simulink model "gm_uz_axi_testIP"  (R2020b)
settings: Solver=FixedStepDiscrete  StartTime=0.0  StopTime=10.0  RelTol=1e-3
settings Model: Creator=ts  LastModifiedBy=ts
settings DataIOCC: LimitDataPoints=on  SaveOutput=off  SaveTime=off
settings OptimizationCC: BlockReduction=off  ConditionallyExecuteInputs=off  DefaultParameterBehavior=Inlined  LifeSpan=inf
settings DebuggingCC: AlgebraicLoopMsg=error  InheritedTsInSrcMsg=none  SingleTaskRateTransMsg=error  AllowSymbolicDim=off  StrictBusMsg=ErrorOnBusTreatedAsVector  SFUnexpectedBacktrackingDiag=warning  SFNoUnconditionalDefaultTransitionDiag=warning  SFExecutionAtInitializationDiag=none  ArithmeticOperatorsInVariantConditions=warning
settings HardwareCC: ProdBitPerPointer=32  ProdBitPerSizeT=32  ProdBitPerPtrDiffT=32  ProdLargestAtomicFloat=None  ProdIntDivRoundTo=Undefined  ProdEndianess=Unspecified  ProdWordSize=32  ProdHWDeviceType=ASIC/FPGA->ASIC/FPGA  ProdEqTarget=off
settings SFSimCC: SimUseLocalCustomCode=off  CustomCodeUndefinedFunction=UseInterfaceOnly
settings RTWCC: RTWUseLocalCustomCode=off
settings CodeAppCC: StateflowObjectComments=on
settings GRTTargetCC: TargetLangStandard=C89/C90 (ANSI)
settings ConfigComp: CovScope=ReferencedModels  CovMetricSettings=dw  CovSaveCumulativeToWorkspaceVar=on  CovSaveSingleToWorkspaceVar=on  CovExternalEMLEnable=off  CovSFcnEnable=off

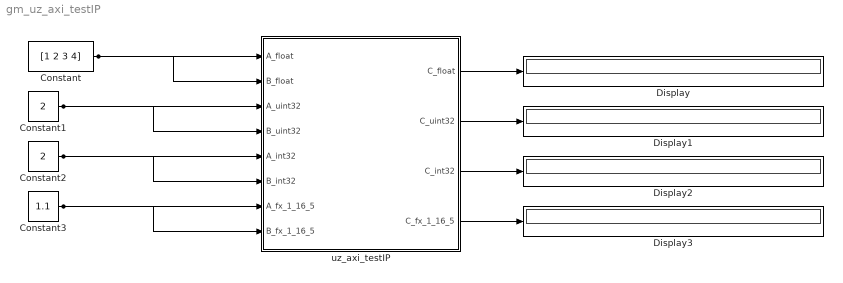
== system gm_uz_axi_testIP ==
  Constant : Constant  Value=[1 2 3 4]  OutDataTypeStr=single  SampleTime=-1
  Constant1 : Constant  Value=2  OutDataTypeStr=uint32  SampleTime=-1
  Constant2 : Constant  Value=2  OutDataTypeStr=int32  SampleTime=-1
  Constant3 : Constant  Value=1.1  OutDataTypeStr=fixdt(1,16,5)  SampleTime=-1
  Display{,1..3} (4 alike) : Display
  uz_axi_testIP : Subsystem  TreatAsAtomicUnit=on
  wires:
  Constant3/1 -> uz_axi_testIP/7(A_fx_1_16_5), uz_axi_testIP/8(B_fx_1_16_5)
  Constant2/1 -> uz_axi_testIP/5(A_int32), uz_axi_testIP/6(B_int32)
  uz_axi_testIP/4(C_fx_1_16_5) -> Display3/1
  uz_axi_testIP/3(C_int32) -> Display2/1
  uz_axi_testIP/2(C_uint32) -> Display1/1
  Constant1/1 -> uz_axi_testIP/3(A_uint32), uz_axi_testIP/4(B_uint32)
  uz_axi_testIP/1(C_float) -> Display/1
  Constant/1 -> uz_axi_testIP/1(A_float), uz_axi_testIP/2(B_float)

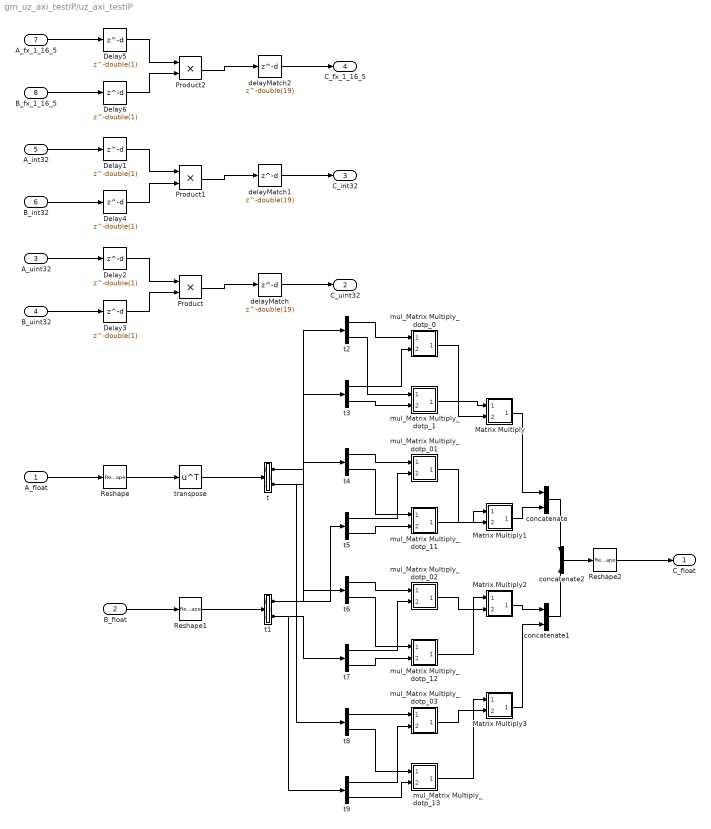
== system gm_uz_axi_testIP/uz_axi_testIP ==
  A_float : Inport  OutDataTypeStr=single  PortDimensions=[4]  SampleTime=0.2
  B_float : Inport  Port=2  OutDataTypeStr=single  PortDimensions=[4]  SampleTime=0.2
  A_uint32 : Inport  Port=3  OutDataTypeStr=uint32  PortDimensions=1  SampleTime=0.2
  B_uint32 : Inport  Port=4  OutDataTypeStr=uint32  PortDimensions=1  SampleTime=0.2
  A_int32 : Inport  Port=5  OutDataTypeStr=int32  PortDimensions=1  SampleTime=0.2
  B_int32 : Inport  Port=6  OutDataTypeStr=int32  PortDimensions=1  SampleTime=0.2
  A_fx_1_16_5 : Inport  Port=7  OutDataTypeStr=fixdt(1, 16, 5)  PortDimensions=1  SampleTime=0.2
  B_fx_1_16_5 : Inport  Port=8  OutDataTypeStr=fixdt(1, 16, 5)  PortDimensions=1  SampleTime=0.2
  Delay{1..6} (6 alike) : Delay  DelayLength=double(1)  InitialCondition=0  SampleTime=0.2
  Matrix Multiply : Subsystem
      mask Display: disp('NFP\nadd');
  Matrix Multiply1 : Subsystem
      mask Display: disp('NFP\nadd');
  Matrix Multiply2 : Subsystem
      mask Display: disp('NFP\nadd');
  Matrix Multiply3 : Subsystem
      mask Display: disp('NFP\nadd');
  Product : Product  Inputs=**  OutDataTypeStr=uint32  SampleTime=0.2
  Product1 : Product  Inputs=**  OutDataTypeStr=int32  SampleTime=0.2
  Product2 : Product  Inputs=**  OutDataTypeStr=fixdt(1, 16, 5)  SampleTime=0.2
  Reshape : Reshape  OutputDimensionality=Customize  OutputDimensions=[2,2]
  Reshape1 : Reshape  OutputDimensionality=Customize  OutputDimensions=[2,2]
  Reshape2 : Reshape  OutputDimensions=[4]
  concatenate : Concatenate
  concatenate1 : Concatenate
  concatenate2 : Concatenate  Mode=Multidimensional array  ConcatenateDimension=2
  delayMatch : Delay  DelayLength=double(19)  InitialCondition=0  SampleTime=0.2
  delayMatch1 : Delay  DelayLength=double(19)  InitialCondition=0  SampleTime=0.2
  delayMatch2 : Delay  DelayLength=double(19)  InitialCondition=0  SampleTime=0.2
  mul_Matrix Multiply_dotp_0 : Subsystem
      mask Display: disp('NFP\nmul');
  mul_Matrix Multiply_dotp_01 : Subsystem
      mask Display: disp('NFP\nmul');
  mul_Matrix Multiply_dotp_02 : Subsystem
      mask Display: disp('NFP\nmul');
  mul_Matrix Multiply_dotp_03 : Subsystem
      mask Display: disp('NFP\nmul');
  mul_Matrix Multiply_dotp_1 : Subsystem
      mask Display: disp('NFP\nmul');
  mul_Matrix Multiply_dotp_11 : Subsystem
      mask Display: disp('NFP\nmul');
  mul_Matrix Multiply_dotp_12 : Subsystem
      mask Display: disp('NFP\nmul');
  mul_Matrix Multiply_dotp_13 : Subsystem
      mask Display: disp('NFP\nmul');
  t : Subsystem
  t1 : Subsystem
  t{2..9} (8 alike) : Demux  Outputs=2
  transpose : Math  Operator=transpose  SaturateOnIntegerOverflow=on
  C_float : Outport  VectorParamsAs1DForOutWhenUnconnected=off
  C_uint32 : Outport  Port=2  VectorParamsAs1DForOutWhenUnconnected=off
  C_int32 : Outport  Port=3  VectorParamsAs1DForOutWhenUnconnected=off
  C_fx_1_16_5 : Outport  Port=4  VectorParamsAs1DForOutWhenUnconnected=off
  wires:
  A_float/1 -> Reshape/1
  B_float/1 -> Reshape1/1
  A_uint32/1 -> Delay2/1
  B_uint32/1 -> Delay3/1
  A_int32/1 -> Delay1/1
  B_int32/1 -> Delay4/1
  A_fx_1_16_5/1 -> Delay5/1
  B_fx_1_16_5/1 -> Delay6/1
  Delay1/1 -> Product1/1
  Delay2/1 -> Product/1
  Delay3/1 -> Product/2
  Delay4/1 -> Product1/2
  Delay5/1 -> Product2/1
  Delay6/1 -> Product2/2
  concatenate2/1 -> Reshape2/1
  delayMatch/1 -> C_uint32/1
  delayMatch1/1 -> C_int32/1
  delayMatch2/1 -> C_fx_1_16_5/1
  Reshape/1 -> transpose/1
  Reshape1/1 -> t1/1(in0)
  Reshape2/1 -> C_float/1
  transpose/1 -> t/1(in0)
  t/1(out0) -> t6/1, t2/1
  t/2(out1) -> t8/1, t4/1
  t1/1(out0) -> t5/1, t3/1
  t1/2(out1) -> t9/1, t7/1
  t2/1 -> mul_Matrix Multiply_dotp_0/1(In1)
  t2/2 -> mul_Matrix Multiply_dotp_1/1(In1)
  t3/1 -> mul_Matrix Multiply_dotp_0/2(In2)
  t3/2 -> mul_Matrix Multiply_dotp_1/2(In2)
  t4/1 -> mul_Matrix Multiply_dotp_01/1(In1)
  t4/2 -> mul_Matrix Multiply_dotp_11/1(In1)
  t5/1 -> mul_Matrix Multiply_dotp_01/2(In2)
  t5/2 -> mul_Matrix Multiply_dotp_11/2(In2)
  concatenate/1 -> concatenate2/1
  t6/1 -> mul_Matrix Multiply_dotp_02/1(In1)
  t6/2 -> mul_Matrix Multiply_dotp_12/1(In1)
  t7/1 -> mul_Matrix Multiply_dotp_02/2(In2)
  t7/2 -> mul_Matrix Multiply_dotp_12/2(In2)
  t8/1 -> mul_Matrix Multiply_dotp_03/1(In1)
  t8/2 -> mul_Matrix Multiply_dotp_13/1(In1)
  t9/1 -> mul_Matrix Multiply_dotp_03/2(In2)
  t9/2 -> mul_Matrix Multiply_dotp_13/2(In2)
  concatenate1/1 -> concatenate2/2
  mul_Matrix Multiply_dotp_0/1(Out1) -> Matrix Multiply/2(In2)
  mul_Matrix Multiply_dotp_1/1(Out1) -> Matrix Multiply/1(In1)
  Matrix Multiply/1(Out1) -> concatenate/1
  mul_Matrix Multiply_dotp_01/1(Out1) -> Matrix Multiply1/2(In2)
  mul_Matrix Multiply_dotp_11/1(Out1) -> Matrix Multiply1/1(In1)
  Matrix Multiply1/1(Out1) -> concatenate/2
  mul_Matrix Multiply_dotp_02/1(Out1) -> Matrix Multiply2/2(In2)
  mul_Matrix Multiply_dotp_12/1(Out1) -> Matrix Multiply2/1(In1)
  Matrix Multiply2/1(Out1) -> concatenate1/1
  mul_Matrix Multiply_dotp_03/1(Out1) -> Matrix Multiply3/2(In2)
  mul_Matrix Multiply_dotp_13/1(Out1) -> Matrix Multiply3/1(In1)
  Matrix Multiply3/1(Out1) -> concatenate1/2
  Product/1 -> delayMatch/1
  Product1/1 -> delayMatch1/1
  Product2/1 -> delayMatch2/1

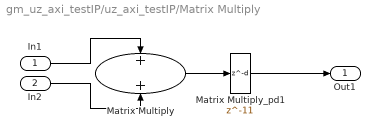
== system gm_uz_axi_testIP/uz_axi_testIP/Matrix Multiply ==
  In1 : Inport
  In2 : Inport  Port=2
  Matrix Multiply : Sum  OutDataTypeStr=single  SampleTime=0.2
  Matrix Multiply_pd1 : Delay  DelayLength=11
  Out1 : Outport
  wires:
  In1/1 -> Matrix Multiply/1
  In2/1 -> Matrix Multiply/2
  Matrix Multiply/1 -> Matrix Multiply_pd1/1
  Matrix Multiply_pd1/1 -> Out1/1

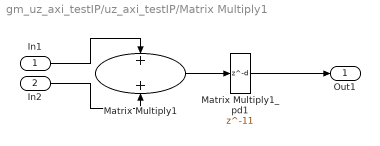
== system gm_uz_axi_testIP/uz_axi_testIP/Matrix Multiply1 ==
  In1 : Inport
  In2 : Inport  Port=2
  Matrix Multiply1 : Sum  OutDataTypeStr=single  SampleTime=0.2
  Matrix Multiply1_pd1 : Delay  DelayLength=11
  Out1 : Outport
  wires:
  In1/1 -> Matrix Multiply1/1
  In2/1 -> Matrix Multiply1/2
  Matrix Multiply1/1 -> Matrix Multiply1_pd1/1
  Matrix Multiply1_pd1/1 -> Out1/1

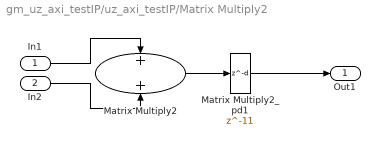
== system gm_uz_axi_testIP/uz_axi_testIP/Matrix Multiply2 ==
  In1 : Inport
  In2 : Inport  Port=2
  Matrix Multiply2 : Sum  OutDataTypeStr=single  SampleTime=0.2
  Matrix Multiply2_pd1 : Delay  DelayLength=11
  Out1 : Outport
  wires:
  In1/1 -> Matrix Multiply2/1
  In2/1 -> Matrix Multiply2/2
  Matrix Multiply2/1 -> Matrix Multiply2_pd1/1
  Matrix Multiply2_pd1/1 -> Out1/1

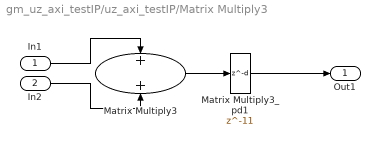
== system gm_uz_axi_testIP/uz_axi_testIP/Matrix Multiply3 ==
  In1 : Inport
  In2 : Inport  Port=2
  Matrix Multiply3 : Sum  OutDataTypeStr=single  SampleTime=0.2
  Matrix Multiply3_pd1 : Delay  DelayLength=11
  Out1 : Outport
  wires:
  In1/1 -> Matrix Multiply3/1
  In2/1 -> Matrix Multiply3/2
  Matrix Multiply3/1 -> Matrix Multiply3_pd1/1
  Matrix Multiply3_pd1/1 -> Out1/1

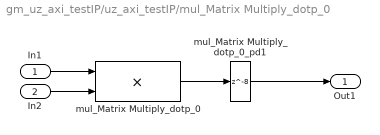
== system gm_uz_axi_testIP/uz_axi_testIP/mul_Matrix Multiply_dotp_0 ==
  In1 : Inport
  In2 : Inport  Port=2
  mul_Matrix Multiply_dotp_0 : Product  Inputs=**  OutDataTypeStr=single  SampleTime=0.2
  mul_Matrix Multiply_dotp_0_pd1 : Delay  DelayLength=8
  Out1 : Outport
  wires:
  In1/1 -> mul_Matrix Multiply_dotp_0/1
  In2/1 -> mul_Matrix Multiply_dotp_0/2
  mul_Matrix Multiply_dotp_0/1 -> mul_Matrix Multiply_dotp_0_pd1/1
  mul_Matrix Multiply_dotp_0_pd1/1 -> Out1/1

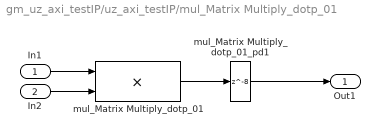
== system gm_uz_axi_testIP/uz_axi_testIP/mul_Matrix Multiply_dotp_01 ==
  In1 : Inport
  In2 : Inport  Port=2
  mul_Matrix Multiply_dotp_01 : Product  Inputs=**  OutDataTypeStr=single  SampleTime=0.2
  mul_Matrix Multiply_dotp_01_pd1 : Delay  DelayLength=8
  Out1 : Outport
  wires:
  In1/1 -> mul_Matrix Multiply_dotp_01/1
  In2/1 -> mul_Matrix Multiply_dotp_01/2
  mul_Matrix Multiply_dotp_01/1 -> mul_Matrix Multiply_dotp_01_pd1/1
  mul_Matrix Multiply_dotp_01_pd1/1 -> Out1/1

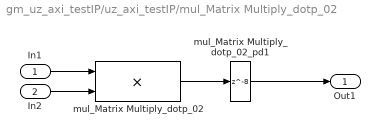
== system gm_uz_axi_testIP/uz_axi_testIP/mul_Matrix Multiply_dotp_02 ==
  In1 : Inport
  In2 : Inport  Port=2
  mul_Matrix Multiply_dotp_02 : Product  Inputs=**  OutDataTypeStr=single  SampleTime=0.2
  mul_Matrix Multiply_dotp_02_pd1 : Delay  DelayLength=8
  Out1 : Outport
  wires:
  In1/1 -> mul_Matrix Multiply_dotp_02/1
  In2/1 -> mul_Matrix Multiply_dotp_02/2
  mul_Matrix Multiply_dotp_02/1 -> mul_Matrix Multiply_dotp_02_pd1/1
  mul_Matrix Multiply_dotp_02_pd1/1 -> Out1/1

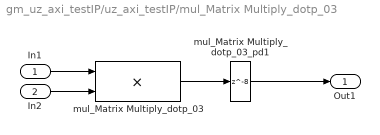
== system gm_uz_axi_testIP/uz_axi_testIP/mul_Matrix Multiply_dotp_03 ==
  In1 : Inport
  In2 : Inport  Port=2
  mul_Matrix Multiply_dotp_03 : Product  Inputs=**  OutDataTypeStr=single  SampleTime=0.2
  mul_Matrix Multiply_dotp_03_pd1 : Delay  DelayLength=8
  Out1 : Outport
  wires:
  In1/1 -> mul_Matrix Multiply_dotp_03/1
  In2/1 -> mul_Matrix Multiply_dotp_03/2
  mul_Matrix Multiply_dotp_03/1 -> mul_Matrix Multiply_dotp_03_pd1/1
  mul_Matrix Multiply_dotp_03_pd1/1 -> Out1/1

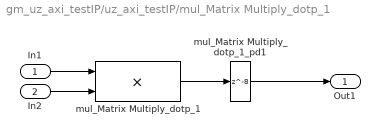
== system gm_uz_axi_testIP/uz_axi_testIP/mul_Matrix Multiply_dotp_1 ==
  In1 : Inport
  In2 : Inport  Port=2
  mul_Matrix Multiply_dotp_1 : Product  Inputs=**  OutDataTypeStr=single  SampleTime=0.2
  mul_Matrix Multiply_dotp_1_pd1 : Delay  DelayLength=8
  Out1 : Outport
  wires:
  In1/1 -> mul_Matrix Multiply_dotp_1/1
  In2/1 -> mul_Matrix Multiply_dotp_1/2
  mul_Matrix Multiply_dotp_1/1 -> mul_Matrix Multiply_dotp_1_pd1/1
  mul_Matrix Multiply_dotp_1_pd1/1 -> Out1/1

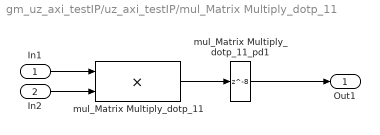
== system gm_uz_axi_testIP/uz_axi_testIP/mul_Matrix Multiply_dotp_11 ==
  In1 : Inport
  In2 : Inport  Port=2
  mul_Matrix Multiply_dotp_11 : Product  Inputs=**  OutDataTypeStr=single  SampleTime=0.2
  mul_Matrix Multiply_dotp_11_pd1 : Delay  DelayLength=8
  Out1 : Outport
  wires:
  In1/1 -> mul_Matrix Multiply_dotp_11/1
  In2/1 -> mul_Matrix Multiply_dotp_11/2
  mul_Matrix Multiply_dotp_11/1 -> mul_Matrix Multiply_dotp_11_pd1/1
  mul_Matrix Multiply_dotp_11_pd1/1 -> Out1/1

== system gm_uz_axi_testIP/uz_axi_testIP/mul_Matrix Multiply_dotp_12 ==
  In1 : Inport
  In2 : Inport  Port=2
  mul_Matrix Multiply_dotp_12 : Product  Inputs=**  OutDataTypeStr=single  SampleTime=0.2
  mul_Matrix Multiply_dotp_12_pd1 : Delay  DelayLength=8
  Out1 : Outport
  wires:
  In1/1 -> mul_Matrix Multiply_dotp_12/1
  In2/1 -> mul_Matrix Multiply_dotp_12/2
  mul_Matrix Multiply_dotp_12/1 -> mul_Matrix Multiply_dotp_12_pd1/1
  mul_Matrix Multiply_dotp_12_pd1/1 -> Out1/1

== system gm_uz_axi_testIP/uz_axi_testIP/mul_Matrix Multiply_dotp_13 ==
  In1 : Inport
  In2 : Inport  Port=2
  mul_Matrix Multiply_dotp_13 : Product  Inputs=**  OutDataTypeStr=single  SampleTime=0.2
  mul_Matrix Multiply_dotp_13_pd1 : Delay  DelayLength=8
  Out1 : Outport
  wires:
  In1/1 -> mul_Matrix Multiply_dotp_13/1
  In2/1 -> mul_Matrix Multiply_dotp_13/2
  mul_Matrix Multiply_dotp_13/1 -> mul_Matrix Multiply_dotp_13_pd1/1
  mul_Matrix Multiply_dotp_13_pd1/1 -> Out1/1

== system gm_uz_axi_testIP/uz_axi_testIP/t ==
  in0 : Inport
  ColVec1 : Selector  NumberOfDimensions=2  IndexOptions=Select all,Index vector (dialog)  Indices=1,1  OutputSizes=1,1
  ColVec2 : Selector  NumberOfDimensions=2  IndexOptions=Select all,Index vector (dialog)  Indices=1,2  OutputSizes=1,1
  out0 : Outport
  out1 : Outport  Port=2
  wires:
  in0/1 -> ColVec1/1, ColVec2/1
  ColVec1/1 -> out0/1
  ColVec2/1 -> out1/1

== system gm_uz_axi_testIP/uz_axi_testIP/t1 ==
  in0 : Inport
  ColVec1 : Selector  NumberOfDimensions=2  IndexOptions=Select all,Index vector (dialog)  Indices=1,1  OutputSizes=1,1
  ColVec2 : Selector  NumberOfDimensions=2  IndexOptions=Select all,Index vector (dialog)  Indices=1,2  OutputSizes=1,1
  out0 : Outport
  out1 : Outport  Port=2
  wires:
  in0/1 -> ColVec1/1, ColVec2/1
  ColVec1/1 -> out0/1
  ColVec2/1 -> out1/1
